simulink model "VSC_GFo_Variable_Frequency_LCL"  (R2017a)
settings: Solver=ode1  StartTime=0.0  StopTime=8  FixedStep=Time_Step  MaxStep=1e-5  RelTol=1e-3
PreLoadFcn:
  | VSC_GFo_Init;
InitFcn:
  | VSC_GFo_Init;
undefined symbols (not defined in the file): GRD00_Lg, GRD00_Rg, Time_Step, VSC01_Delta_P_Time_Step, VSC01_Delta_P_Value
libraries: powerlib x7, Source_Lib x1, GFo_Lib x1
settings Model: Creator=Frederic_Colas  LastModifiedBy=fcolas
settings OptimizationCC: LifeSpan=inf
settings DebuggingCC: UnconnectedInputMsg=none  UnconnectedOutputMsg=none  UnconnectedLineMsg=none  SFExecutionAtInitializationDiag=none
settings HardwareCC: ProdBitPerSizeT=32  ProdBitPerPtrDiffT=32  ProdWordSize=32  ProdHWDeviceType=Specified
settings SimscapeCC: SimscapeNormalizeSystem=off

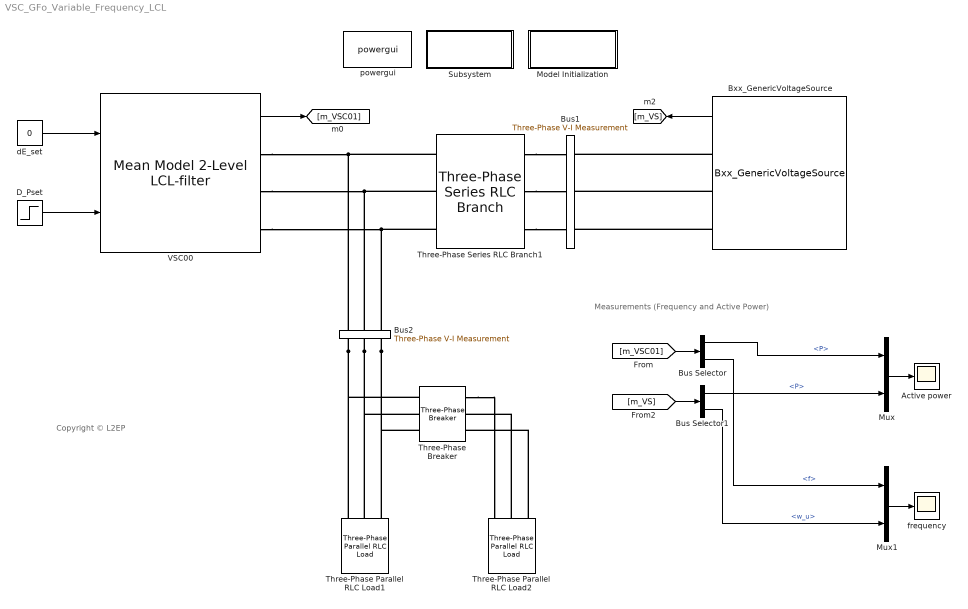
== system VSC_GFo_Variable_Frequency_LCL ==
  note: Measurements (Frequency and Active Power)
  note: Copyright © L2EP
  Active power : Scope
  Bus Selector : BusSelector  OutputSignals=control.P,control.f
  Bus Selector1 : BusSelector  OutputSignals=P,w_u
  Bus1 : powerlib/Measurements/Three-Phase V-I Measurement  VoltageMeasurement=no  SetLabelV=off  LabelV=Vabc  Vpu=off  VpuLL=off  CurrentMeasurement=no  SetLabelI=off  LabelI=Iabc  Ipu=off  Pbase=1e9  Vbase=VSC01_Un2  OutputType=Complex  PhasorSimulation=off  PSBequivalent=0
  "Bus2 " : powerlib/Measurements/Three-Phase V-I Measurement  VoltageMeasurement=no  SetLabelV=off  LabelV=Vabc  Vpu=off  VpuLL=off  CurrentMeasurement=no  SetLabelI=off  LabelI=Iabc  Ipu=off  Pbase=100e6  Vbase=500e3  OutputType=Complex  PhasorSimulation=off  PSBequivalent=0
  Bxx_GenericVoltageSource : Source_Lib/Bxx_GenericVoltageSource  SourceNature_str=INERTIAL  fn=fb  Sn=1e9  Un=GRD00_Un  LFpopup=Swing  P0=-398686071.6266  Q0=7934005.2103  V0_pu=1  U0=20000  Theta0_deg=0  H_s=GRD00_H  DroopOnOff=on  R_percent=GRD00_R  TN=GRD00_TN  TD=GRD00_TD
      settings: SourceProductName=VSC4SPS
  D_Pset : Step  Time=VSC01_Delta_P_Time_Step  After=VSC01_Delta_P_Value  SampleTime=0
  Model Initialization : Subsystem  mask(Model Functions){InitFcnX=VSC_GFo_Init;, prel=on, posl=off, inif=on, strf=off}
      mask prompts: InitFcnX "Initialisation"; prel "Preload Function"; posl "PostLoad Function"; inif "InitFcn"; strf "StartFcn"
      mask init:
      | currentBlock = gcb;
      | root = bdroot(currentBlock);
      | 
      | if ~strcmp(get_param(root,'BlockDiagramType'),'library')
      |     if prel==1
      |         set_param(root, 'PreLoadFcn', InitFcnX);
      |     else
      |         set_param(root, 'PreLoadFcn', '');
      |     end
      |     if inif==1
      |         set_param(root, 'InitFcn', InitFcnX);
      |     else
      |         set_param(root, 'InitFcn', '');
      |     end
      |     if strf==1
      |         set_param(root, 'StartFcn', InitFcnX);
      |     else
      |         set_param(root, 'StartFcn', '');
      |     end
      |     if posl==1
      |         set_param(root, 'PostLoadFcn', InitFcnX);
      |     else
      |         set_param(root, 'PostLoadFcn', '');
      |     end
      | end
      | 
      | pos = get_param(currentBlock, 'Position');
      | width = pos(3) - pos(1); height = pos(4) - pos(2);
      | txt = [ upper(root) '\n' '- InitFcn. . . . . '  get_param(root, 'InitFcn') ];
      settings: CopyFcn=set_param(gcb,'LinkStatus','none')
      mask Display:
      | %text(5, height*0.5, txt, 'horizontalAlignment', 'left', 'verticalAlignment', 'middle') ;
      | color('blue'),disp('Initialization Function\nParameters')
  Mux : Mux  Inputs=2
  Mux1 : Mux  Inputs=2
  Subsystem : Subsystem
      settings: OpenFcn=LoadFlow_VSC
      mask Display: color('blue'),disp('Update Loadflow')
  Three-Phase Parallel RLC Load1 : powerlib/Elements/Three-Phase Parallel RLC Load  LConnTagsString=A|B|C  Configuration=Y (grounded)  NominalVoltage=GRD00_Un  Vabc=[1e3 1e3 1e3]  Vabcp=[1e3 1e3 1e3]  NominalFrequency=fb  UnbalancedPower=off  ActivePower=100e6  InductivePower=0  CapacitivePower=0  Pabc=[10e3 9e3 11e3]  QLabc=[100 90 110]  QCabc=[100 90 110]  Pabcp=[10e3 9e3 11e3]  QLabcp=[100 90 110]  QCabcp=[100 90 110]  Measurements=None  LoadType=constant Z
  Three-Phase Parallel RLC Load2 : powerlib/Elements/Three-Phase Parallel RLC Load  LConnTagsString=A|B|C  Configuration=Y (grounded)  NominalVoltage=GRD00_Un  Vabc=[1e3 1e3 1e3]  Vabcp=[1e3 1e3 1e3]  NominalFrequency=fb  UnbalancedPower=off  ActivePower=400e6  InductivePower=0  CapacitivePower=0  Pabc=[10e3 9e3 11e3]  QLabc=[100 90 110]  QCabc=[100 90 110]  Pabcp=[10e3 9e3 11e3]  QLabcp=[100 90 110]  QCabcp=[100 90 110]  Measurements=None  LoadType=constant Z
  Three-Phase Series RLC Branch1 : powerlib/Elements/Three-Phase Series RLC Branch  LConnTagsString=A|B|C  RConnTagsString=A|B|C  BranchType=RL  Resistance=GRD00_Rg  Inductance=GRD00_Lg  Capacitance=1e-6  Measurements=None
  Three-Phase Breaker : powerlib/Elements/Three-Phase Breaker  InitialState=open  SwitchA=on  SwitchB=on  SwitchC=on  SwitchTimes=[1 60]  External=off  BreakerResistance=0.01  SnubberResistance=1e6  SnubberCapacitance=inf  Measurements=None
  VSC00 : GFo_Lib/Mean Model 2-Level LCL-filter  fn=fn  Sn=VSC01_Sn  Pn=VSC01_Pn  Udcn=VSC01_Udc_n  Un1=VSC01_Un1  Un2=VSC01_Un2  Rt_pu=VSC01_Rt_pu  Lt_pu=VSC01_Lt_pu  Rm_pu=500  Lm_pu=500  Lf_pu=VSC01_Lf_pu  Rf_pu=VSC01_Rf_pu  Cf_pu=VSC01_Cf_pu  Tr_PLL=VSC01_Tr_PLL  Val_Freq_Support=on  Val_gamma=on  R_percent=VSC01_R  Rv=VSC01_Rv  W_TVR=VSC01_W_LF  I_thresh_pu=1  DX_DR=5  Kp_Rvi_pu=0.676  gainpopup=3  wc1=VSC01_wc1  mp1=VSC01_mp1  wc2=VSC01_wc2  mp2=VSC01_mp2  wc3=VSC01_wc3  mp3=VSC01_mp3  T1=VSC01_T1  T2=VSC01_T2  LFpopup=PQ  P0=0.5  Q0=1.6671e-05  V0=1.0018  Theta0=1.1424  innercontrol=1  Kp_i=0.73  Ki_i=1.19  Kp_v=0.52  Ki_v=1.16  Kffv=1  Kffi=1  I_max=1.25
      settings: SourceProductName=VSC4SPS
  dE_set : Constant  Value=0
  frequency : Scope
  powergui : powerlib/powergui  Priority=1  SimulationMode=Discrete  SampleTime=Time_Step  frequency=60  Iterations=50  frequencyindice=50  Pbase=1000000000  ErrMax=1e-4  UnitsV=kV  UnitsW=MW  buscounter=0  FunctionMessages=off  echomessages=off  EnableUseOfTLC=off  CurrentSourceSwitches=off  DisableSnubberDevices=off  DisableRonSwitches=off  DisableVfSwitches=off  DisplayEquations=off  SolverType=Tustin/Backward Euler (TBE)  Interpol=off  ExternalGateDelay=off  methode=off  Ts=100  x0status=blocks  SPID=on  SwTol=0  HookPort=off  RestoreLinks=warning  ResistiveCurrentMeasurement=off  Frange=[0:2:500]  Ylog=off  Xlog=on  ShowGrid=off  save=off  variable=ZData  structure=0  ZoomFFT=off  StartTime=0.0  cycles=1  DisplayStyle=1  fundamental=60  FreqAxis=off  MaxFrequency=1000  frequencyindicesteady=1  RmsSteady=1  display=off
  wires:
  VSC00/1 -> [m_VSC01]
  Bxx_GenericVoltageSource/1 -> [m_VS]
  Mux1/1 -> frequency/1
  [m_VS] -> Bus Selector1/1
  [m_VSC01] -> Bus Selector/1
  Bus Selector1/2 -> Mux1/2  "<w_u>"
  Mux/1 -> Active power/1
  Bus Selector1/1 -> Mux/2  "<P>"
  Bus Selector/2 -> Mux1/1  "<f>"
  Bus Selector/1 -> Mux/1  "<P>"
  D_Pset/1 -> VSC00/2
  dE_set/1 -> VSC00/1
  connections:
  Three-Phase Series RLC Branch1/LConn1 -- VSC00/RConn1 -- "Bus2 "/LConn3
  Three-Phase Series RLC Branch1/RConn2 -- Bus1/LConn2
  Three-Phase Series RLC Branch1/LConn3 -- VSC00/RConn3 -- "Bus2 "/LConn1
  Three-Phase Series RLC Branch1/LConn2 -- VSC00/RConn2 -- "Bus2 "/LConn2
  Three-Phase Series RLC Branch1/RConn3 -- Bus1/LConn3
  Three-Phase Series RLC Branch1/RConn1 -- Bus1/LConn1
  Bxx_GenericVoltageSource/RConn1 -- Bus1/RConn1
  Bxx_GenericVoltageSource/RConn2 -- Bus1/RConn2
  Bxx_GenericVoltageSource/RConn3 -- Bus1/RConn3
  "Bus2 "/RConn1 -- Three-Phase Breaker/LConn3 -- Three-Phase Parallel RLC Load1/LConn3
  "Bus2 "/RConn3 -- Three-Phase Breaker/LConn1 -- Three-Phase Parallel RLC Load1/LConn1
  "Bus2 "/RConn2 -- Three-Phase Breaker/LConn2 -- Three-Phase Parallel RLC Load1/LConn2
  Three-Phase Breaker/RConn1 -- Three-Phase Parallel RLC Load2/LConn1
  Three-Phase Parallel RLC Load2/LConn3 -- Three-Phase Breaker/RConn3
  Three-Phase Parallel RLC Load2/LConn2 -- Three-Phase Breaker/RConn2

== system VSC_GFo_Variable_Frequency_LCL/Model Initialization ==

== system VSC_GFo_Variable_Frequency_LCL/Subsystem ==
